simulink model "gm_dvfs_zed_simple_backup"  (R2025b)
settings: Solver=FixedStepDiscrete  StartTime=0.0  StopTime=10.0  FixedStep=0.1  RelTol=1e-3
libraries: simulink x6
settings Model: Creator=Vimal Rency  LastModifiedBy=Vimal Rency
settings OptimizationCC: BlockReduction=off  ConditionallyExecuteInputs=off
settings DebuggingCC: InheritedTsInSrcMsg=none

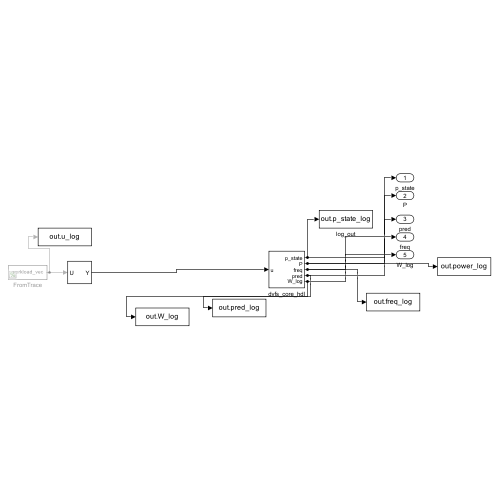
[thumbnail: Simulink's stored preview of the top-level diagram]
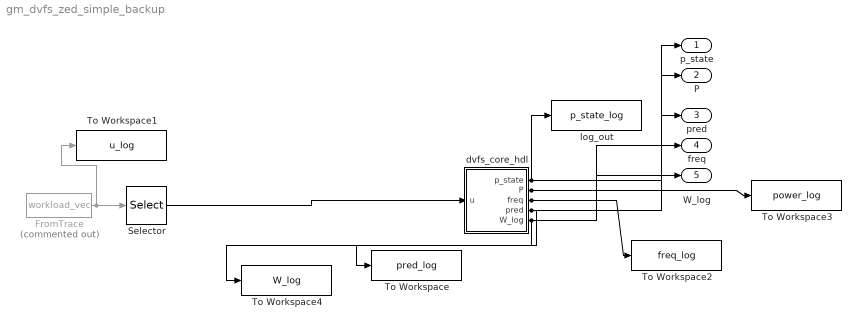
== system gm_dvfs_zed_simple_backup ==
  FromTrace : FromWorkspace  Commented=on  VariableName=workload_vec
  Selector : Selector  NumberOfDimensions=2  InputPortWidth=3  IndexOptions=Select all,Index vector (dialog)  Indices=[1 3],1  OutputSizes=1,1
  To Workspace : ToWorkspace  VariableName=pred_log  SampleTime=-1
  To Workspace1 : ToWorkspace  VariableName=u_log  SampleTime=-1
  To Workspace2 : ToWorkspace  VariableName=freq_log  SampleTime=-1
  To Workspace3 : ToWorkspace  VariableName=power_log  SampleTime=-1
  To Workspace4 : ToWorkspace  VariableName=W_log  SampleTime=-1
  dvfs_core_hdl : Subsystem
  log_out : ToWorkspace  VariableName=p_state_log  SampleTime=-1
  p_state : Outport
  P : Outport  Port=2
  pred : Outport  Port=3
  freq : Outport  Port=4
  W_log : Outport  Port=5
  wires:
  dvfs_core_hdl/5(W_log) -> To Workspace4/1, W_log/1
  dvfs_core_hdl/4(pred) -> To Workspace/1, pred/1
  dvfs_core_hdl/3(freq) -> To Workspace2/1, freq/1
  dvfs_core_hdl/2(P) -> To Workspace3/1, P/1
  dvfs_core_hdl/1(p_state) -> log_out/1, p_state/1
  Selector/1 -> dvfs_core_hdl/1(u)
  FromTrace/1 -> Selector/1, To Workspace1/1

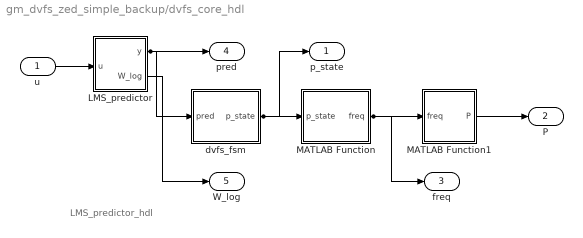
== system gm_dvfs_zed_simple_backup/dvfs_core_hdl ==
  note: LMS_predictor_hdl
  u : Inport  OutDataTypeStr=double  PortDimensions=1  SampleTime=0.1
  LMS_predictor : Subsystem
  MATLAB Function : Subsystem
  MATLAB Function1 : Subsystem
  dvfs_fsm : Subsystem
  p_state : Outport  SampleTime=0.1
  P : Outport  Port=2  SampleTime=0.1
  freq : Outport  Port=3  SampleTime=0.1
  pred : Outport  Port=4  SampleTime=0.1
  W_log : Outport  Port=5  SampleTime=0.1
  wires:
  u/1 -> LMS_predictor/1(u)
  dvfs_fsm/1(p_state) -> MATLAB Function/1(p_state), p_state/1
  LMS_predictor/1(y) -> dvfs_fsm/1(pred), pred/1
  LMS_predictor/2(W_log) -> W_log/1
  MATLAB Function/1(freq) -> MATLAB Function1/1(freq), freq/1
  MATLAB Function1/1(P) -> P/1

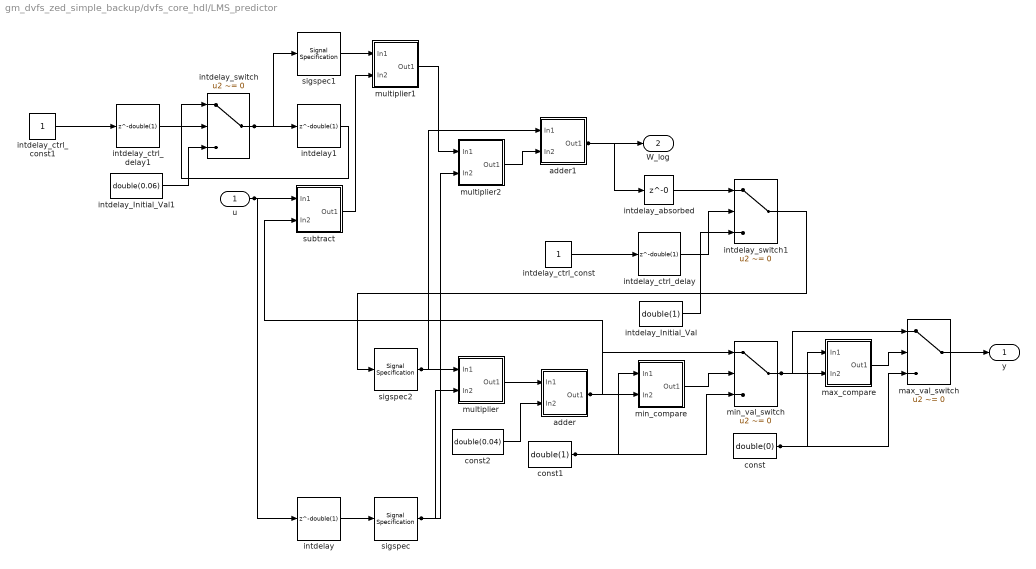
== system gm_dvfs_zed_simple_backup/dvfs_core_hdl/LMS_predictor ==
  u : Inport  OutDataTypeStr=double  PortDimensions=1  SampleTime=0.1
  adder : Subsystem
      mask Display: disp('NFP\nadd');
  adder1 : Subsystem
      mask Display: disp('NFP\nadd');
  const : Constant  Value=double(0)  VectorParams1D=off  OutDataTypeStr=double  SampleTime=0.1
  const1 : Constant  Value=double(1)  VectorParams1D=off  OutDataTypeStr=double  SampleTime=0.1
  const2 : Constant  Value=double(0.04)  VectorParams1D=off  OutDataTypeStr=double  SampleTime=0.1
  intdelay : Delay  DelayLength=double(1)  InitialCondition=0  SampleTime=0.1
  intdelay1 : Delay  DelayLength=double(1)  InitialCondition=0  SampleTime=0.1
  intdelay_Initial_Val : Constant  Value=double(1)  OutDataTypeStr=double  SampleTime=0.1
  intdelay_Initial_Val1 : Constant  Value=double(0.06)  OutDataTypeStr=double  SampleTime=0.1
  intdelay_absorbed : Delay  DelayLength=0
  intdelay_ctrl_const : Constant  OutDataTypeStr=boolean  SampleTime=0.1
  intdelay_ctrl_const1 : Constant  OutDataTypeStr=boolean  SampleTime=0.1
  intdelay_ctrl_delay : Delay  DelayLength=double(1)  InitialCondition=0  SampleTime=0.1
  intdelay_ctrl_delay1 : Delay  DelayLength=double(1)  InitialCondition=0  SampleTime=0.1
  intdelay_switch : Switch  Criteria=u2 ~= 0  Threshold=double(0)  OutDataTypeStr=double  SampleTime=0.1  SaturateOnIntegerOverflow=off  InputSameDT=off
  intdelay_switch1 : Switch  Criteria=u2 ~= 0  Threshold=double(0)  OutDataTypeStr=double  SampleTime=0.1  SaturateOnIntegerOverflow=off  InputSameDT=off
  max_compare : Subsystem
      mask Display: disp('NFP\nrelop');
  max_val_switch : Switch  Criteria=u2 ~= 0  Threshold=double(0)  OutDataTypeStr=double  SampleTime=0.1  SaturateOnIntegerOverflow=off  InputSameDT=off
  min_compare : Subsystem
      mask Display: disp('NFP\nrelop');
  min_val_switch : Switch  Criteria=u2 ~= 0  Threshold=double(0)  OutDataTypeStr=double  SampleTime=0.1  SaturateOnIntegerOverflow=off  InputSameDT=off
  multiplier : Subsystem
      mask Display: disp('NFP\nmul');
  multiplier1 : Subsystem
      mask Display: disp('NFP\nmul');
  multiplier2 : Subsystem
      mask Display: disp('NFP\nmul');
  sigspec : SignalSpecification  OutDataTypeStr=double  Dimensions=1
  sigspec1 : SignalSpecification  OutDataTypeStr=double  Dimensions=1
  sigspec2 : SignalSpecification  OutDataTypeStr=double  Dimensions=1
  subtract : Subsystem
      mask Display: disp('NFP\nadd');
  y : Outport  SampleTime=0.1
  W_log : Outport  Port=2  SampleTime=0.1
  wires:
  sigspec1/1 -> multiplier1/1(In1)
  u/1 -> intdelay/1, subtract/1(In1)
  multiplier1/1(Out1) -> multiplier2/1(In1)
  intdelay_ctrl_const1/1 -> intdelay_ctrl_delay1/1
  intdelay1/1 -> intdelay_switch/1
  sigspec2/1 -> adder1/1(In1), multiplier/1(In1)
  intdelay_ctrl_delay1/1 -> intdelay_switch/2
  intdelay_Initial_Val1/1 -> intdelay_switch/3
  intdelay_switch1/1 -> sigspec2/1
  intdelay_switch/1 -> sigspec1/1, intdelay1/1
  subtract/1(Out1) -> multiplier1/2(In2)
  intdelay/1 -> sigspec/1
  sigspec/1 -> multiplier/2(In2), multiplier2/2(In2)
  intdelay_ctrl_delay/1 -> intdelay_switch1/2
  multiplier2/1(Out1) -> adder1/2(In2)
  multiplier/1(Out1) -> adder/1(In1)
  const2/1 -> adder/2(In2)
  adder1/1(Out1) -> intdelay_absorbed/1, W_log/1
  intdelay_ctrl_const/1 -> intdelay_ctrl_delay/1
  adder/1(Out1) -> min_val_switch/1, min_compare/2(In2), subtract/2(In2)
  const1/1 -> min_val_switch/3, min_compare/1(In1)
  intdelay_absorbed/1 -> intdelay_switch1/1
  intdelay_Initial_Val/1 -> intdelay_switch1/3
  min_compare/1(Out1) -> min_val_switch/2
  min_val_switch/1 -> max_val_switch/1, max_compare/2(In2)
  const/1 -> max_val_switch/3, max_compare/1(In1)
  max_compare/1(Out1) -> max_val_switch/2
  max_val_switch/1 -> y/1

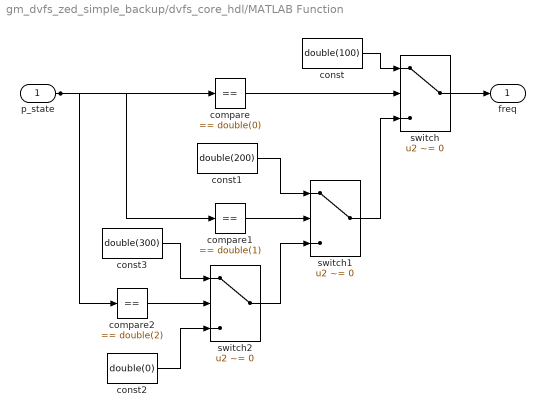
== system gm_dvfs_zed_simple_backup/dvfs_core_hdl/MATLAB Function ==
  p_state : Inport  OutDataTypeStr=uint8  PortDimensions=1  SampleTime=0.1
  compare : simulink/Logic and Bit Operations/Compare To Constant  relop===  const=double(0)  OutDataTypeStr=boolean
  compare1 : simulink/Logic and Bit Operations/Compare To Constant  relop===  const=double(1)  OutDataTypeStr=boolean
  compare2 : simulink/Logic and Bit Operations/Compare To Constant  relop===  const=double(2)  OutDataTypeStr=boolean
  const : Constant  Value=double(100)  VectorParams1D=off  OutDataTypeStr=double  SampleTime=0.1
  const1 : Constant  Value=double(200)  VectorParams1D=off  OutDataTypeStr=double  SampleTime=0.1
  const2 : Constant  Value=double(0)  VectorParams1D=off  OutDataTypeStr=double  SampleTime=0.1
  const3 : Constant  Value=double(300)  VectorParams1D=off  OutDataTypeStr=double  SampleTime=0.1
  switch : Switch  Criteria=u2 ~= 0  Threshold="fi(0,0,1,0,\"hex\",\"0\")"  OutDataTypeStr=double  SampleTime=0.1  SaturateOnIntegerOverflow=off  InputSameDT=off
  switch1 : Switch  Criteria=u2 ~= 0  Threshold="fi(0,0,1,0,\"hex\",\"0\")"  OutDataTypeStr=double  SampleTime=0.1  SaturateOnIntegerOverflow=off  InputSameDT=off
  switch2 : Switch  Criteria=u2 ~= 0  Threshold="fi(0,0,1,0,\"hex\",\"0\")"  OutDataTypeStr=double  SampleTime=0.1  SaturateOnIntegerOverflow=off  InputSameDT=off
  freq : Outport  SampleTime=0.1
  wires:
  const2/1 -> switch2/3
  p_state/1 -> compare1/1, compare/1, compare2/1
  const3/1 -> switch2/1
  switch2/1 -> switch1/3
  compare2/1 -> switch2/2
  compare/1 -> switch/2
  const1/1 -> switch1/1
  compare1/1 -> switch1/2
  const/1 -> switch/1
  switch1/1 -> switch/3
  switch/1 -> freq/1

== system gm_dvfs_zed_simple_backup/dvfs_core_hdl/MATLAB Function1 ==
  freq : Inport  OutDataTypeStr=double  PortDimensions=1  SampleTime=0.1
  gain : Subsystem
      mask Display: disp('NFP\nmul');
  gain_const : Constant  Value=double(0.01)  OutDataTypeStr=double  SampleTime=0.1
  P : Outport  SampleTime=0.1
  wires:
  gain/1(Out1) -> P/1
  gain_const/1 -> gain/1(In1)
  freq/1 -> gain/2(In2)

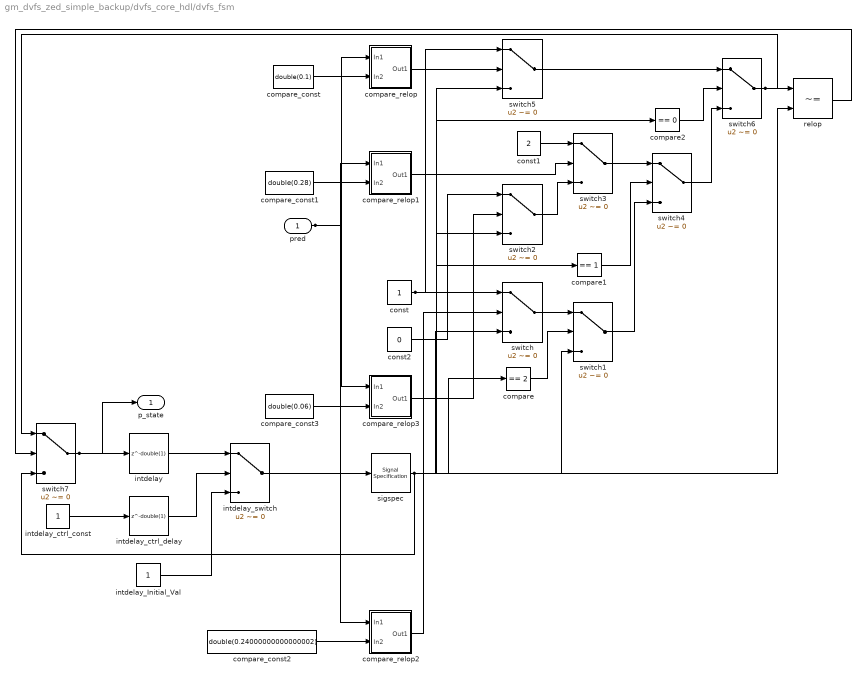
== system gm_dvfs_zed_simple_backup/dvfs_core_hdl/dvfs_fsm ==
  pred : Inport  OutDataTypeStr=double  PortDimensions=1  SampleTime=0.1
  compare : simulink/Logic and Bit Operations/Compare To Constant  relop===  const=2  OutDataTypeStr=boolean
  compare1 : simulink/Logic and Bit Operations/Compare To Constant  relop===  const=1  OutDataTypeStr=boolean
  compare2 : simulink/Logic and Bit Operations/Compare To Constant  relop===  const=0  OutDataTypeStr=boolean
  compare_const : Constant  Value=double(0.1)  OutDataTypeStr=double  SampleTime=0.1
  compare_const1 : Constant  Value=double(0.28)  OutDataTypeStr=double  SampleTime=0.1
  compare_const2 : Constant  Value=double(0.24000000000000002)  OutDataTypeStr=double  SampleTime=0.1
  compare_const3 : Constant  Value=double(0.06)  OutDataTypeStr=double  SampleTime=0.1
  compare_relop : Subsystem
      mask Display: disp('NFP\nrelop');
  compare_relop1 : Subsystem
      mask Display: disp('NFP\nrelop');
  compare_relop2 : Subsystem
      mask Display: disp('NFP\nrelop');
  compare_relop3 : Subsystem
      mask Display: disp('NFP\nrelop');
  const : Constant  VectorParams1D=off  OutDataTypeStr=uint8  SampleTime=0.1
  const1 : Constant  Value=2  VectorParams1D=off  OutDataTypeStr=uint8  SampleTime=0.1
  const2 : Constant  Value=0  VectorParams1D=off  OutDataTypeStr=uint8  SampleTime=0.1
  intdelay : Delay  DelayLength=double(1)  InitialCondition=0  SampleTime=0.1
  intdelay_Initial_Val : Constant  OutDataTypeStr=uint8  SampleTime=0.1
  intdelay_ctrl_const : Constant  OutDataTypeStr=boolean  SampleTime=0.1
  intdelay_ctrl_delay : Delay  DelayLength=double(1)  InitialCondition=0  SampleTime=0.1
  intdelay_switch : Switch  Criteria=u2 ~= 0  Threshold=double(0)  OutDataTypeStr=uint8  SampleTime=0.1  SaturateOnIntegerOverflow=off  InputSameDT=off
  relop : RelationalOperator  Operator=~=  OutDataTypeStr=boolean  SampleTime=0.1  InputSameDT=off
  sigspec : SignalSpecification  OutDataTypeStr=uint8  Dimensions=1
  switch{,1..7} (8 alike) : Switch  Criteria=u2 ~= 0  Threshold="fi(0,0,1,0,\"hex\",\"0\")"  OutDataTypeStr=uint8  SampleTime=0.1  SaturateOnIntegerOverflow=off  InputSameDT=off
  p_state : Outport  SampleTime=0.1
  wires:
  switch7/1 -> p_state/1, intdelay/1
  intdelay_Initial_Val/1 -> intdelay_switch/3
  intdelay_ctrl_const/1 -> intdelay_ctrl_delay/1
  sigspec/1 -> switch7/3, switch1/3, compare2/1, relop/2, compare1/1, switch2/3, switch/3, compare/1, switch5/3
  compare_const/1 -> compare_relop/2(In2)
  intdelay/1 -> intdelay_switch/1
  compare_const1/1 -> compare_relop1/2(In2)
  intdelay_ctrl_delay/1 -> intdelay_switch/2
  pred/1 -> compare_relop1/1(In1), compare_relop/1(In1), compare_relop2/1(In1), compare_relop3/1(In1)
  compare_relop2/1(Out1) -> switch/2
  compare_const3/1 -> compare_relop3/2(In2)
  intdelay_switch/1 -> sigspec/1
  switch1/1 -> switch4/3
  compare_const2/1 -> compare_relop2/2(In2)
  const1/1 -> switch3/1
  compare_relop/1(Out1) -> switch5/2
  compare_relop1/1(Out1) -> switch3/2
  const/1 -> switch5/1, switch/1
  const2/1 -> switch2/1
  compare_relop3/1(Out1) -> switch2/2
  switch5/1 -> switch6/1
  switch2/1 -> switch3/3
  switch/1 -> switch1/1
  compare/1 -> switch1/2
  switch3/1 -> switch4/1
  compare1/1 -> switch4/2
  compare2/1 -> switch6/2
  switch4/1 -> switch6/3
  switch6/1 -> switch7/1, relop/1
  relop/1 -> switch7/2

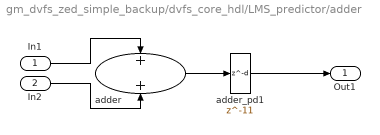
== system gm_dvfs_zed_simple_backup/dvfs_core_hdl/LMS_predictor/adder ==
  In1 : Inport
  In2 : Inport  Port=2
  adder : Sum  OutDataTypeStr=double  SampleTime=0.1
  adder_pd1 : Delay  DelayLength=11
  Out1 : Outport
  wires:
  In1/1 -> adder/1
  In2/1 -> adder/2
  adder/1 -> adder_pd1/1
  adder_pd1/1 -> Out1/1

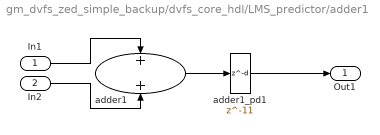
== system gm_dvfs_zed_simple_backup/dvfs_core_hdl/LMS_predictor/adder1 ==
  In1 : Inport
  In2 : Inport  Port=2
  adder1 : Sum  OutDataTypeStr=double  SampleTime=0.1
  adder1_pd1 : Delay  DelayLength=11
  Out1 : Outport
  wires:
  In1/1 -> adder1/1
  In2/1 -> adder1/2
  adder1/1 -> adder1_pd1/1
  adder1_pd1/1 -> Out1/1

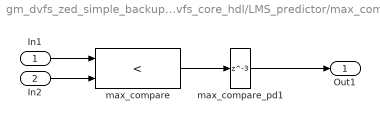
== system gm_dvfs_zed_simple_backup/dvfs_core_hdl/LMS_predictor/max_compare ==
  In1 : Inport
  In2 : Inport  Port=2
  max_compare : RelationalOperator  Operator=<  OutDataTypeStr=boolean  SampleTime=0.1
  max_compare_pd1 : Delay  DelayLength=3
  Out1 : Outport
  wires:
  In1/1 -> max_compare/1
  In2/1 -> max_compare/2
  max_compare/1 -> max_compare_pd1/1
  max_compare_pd1/1 -> Out1/1

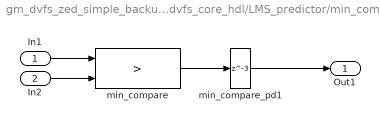
== system gm_dvfs_zed_simple_backup/dvfs_core_hdl/LMS_predictor/min_compare ==
  In1 : Inport
  In2 : Inport  Port=2
  min_compare : RelationalOperator  Operator=>  OutDataTypeStr=boolean  SampleTime=0.1
  min_compare_pd1 : Delay  DelayLength=3
  Out1 : Outport
  wires:
  In1/1 -> min_compare/1
  In2/1 -> min_compare/2
  min_compare/1 -> min_compare_pd1/1
  min_compare_pd1/1 -> Out1/1

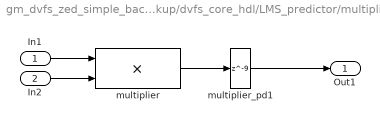
== system gm_dvfs_zed_simple_backup/dvfs_core_hdl/LMS_predictor/multiplier ==
  In1 : Inport
  In2 : Inport  Port=2
  multiplier : Product  Inputs=**  OutDataTypeStr=double  SampleTime=0.1
  multiplier_pd1 : Delay  DelayLength=9
  Out1 : Outport
  wires:
  In1/1 -> multiplier/1
  In2/1 -> multiplier/2
  multiplier/1 -> multiplier_pd1/1
  multiplier_pd1/1 -> Out1/1

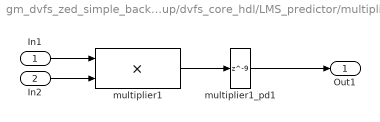
== system gm_dvfs_zed_simple_backup/dvfs_core_hdl/LMS_predictor/multiplier1 ==
  In1 : Inport
  In2 : Inport  Port=2
  multiplier1 : Product  Inputs=**  OutDataTypeStr=double  SampleTime=0.1
  multiplier1_pd1 : Delay  DelayLength=9
  Out1 : Outport
  wires:
  In1/1 -> multiplier1/1
  In2/1 -> multiplier1/2
  multiplier1/1 -> multiplier1_pd1/1
  multiplier1_pd1/1 -> Out1/1

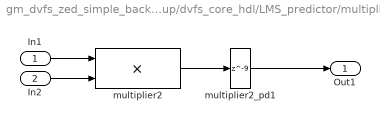
== system gm_dvfs_zed_simple_backup/dvfs_core_hdl/LMS_predictor/multiplier2 ==
  In1 : Inport
  In2 : Inport  Port=2
  multiplier2 : Product  Inputs=**  OutDataTypeStr=double  SampleTime=0.1
  multiplier2_pd1 : Delay  DelayLength=9
  Out1 : Outport
  wires:
  In1/1 -> multiplier2/1
  In2/1 -> multiplier2/2
  multiplier2/1 -> multiplier2_pd1/1
  multiplier2_pd1/1 -> Out1/1

== system gm_dvfs_zed_simple_backup/dvfs_core_hdl/LMS_predictor/subtract ==
  In1 : Inport
  In2 : Inport  Port=2
  subtract : Sum  Inputs=+-  OutDataTypeStr=double  SampleTime=0.1
  subtract_pd1 : Delay  DelayLength=11
  Out1 : Outport
  wires:
  In1/1 -> subtract/1
  In2/1 -> subtract/2
  subtract/1 -> subtract_pd1/1
  subtract_pd1/1 -> Out1/1

== system gm_dvfs_zed_simple_backup/dvfs_core_hdl/MATLAB Function1/gain ==
  In1 : Inport
  In2 : Inport  Port=2
  gain : Product  Inputs=**  OutDataTypeStr=double  SampleTime=0.1
  gain_pd1 : Delay  DelayLength=9
  Out1 : Outport
  wires:
  In1/1 -> gain/1
  In2/1 -> gain/2
  gain/1 -> gain_pd1/1
  gain_pd1/1 -> Out1/1

== system gm_dvfs_zed_simple_backup/dvfs_core_hdl/dvfs_fsm/compare_relop ==
  In1 : Inport
  In2 : Inport  Port=2
  compare_relop : RelationalOperator  OutDataTypeStr=boolean  SampleTime=0.1
  compare_relop_pd1 : Delay  DelayLength=3
  Out1 : Outport
  wires:
  In1/1 -> compare_relop/1
  In2/1 -> compare_relop/2
  compare_relop/1 -> compare_relop_pd1/1
  compare_relop_pd1/1 -> Out1/1

== system gm_dvfs_zed_simple_backup/dvfs_core_hdl/dvfs_fsm/compare_relop1 ==
  In1 : Inport
  In2 : Inport  Port=2
  compare_relop1 : RelationalOperator  OutDataTypeStr=boolean  SampleTime=0.1
  compare_relop1_pd1 : Delay  DelayLength=3
  Out1 : Outport
  wires:
  In1/1 -> compare_relop1/1
  In2/1 -> compare_relop1/2
  compare_relop1/1 -> compare_relop1_pd1/1
  compare_relop1_pd1/1 -> Out1/1

== system gm_dvfs_zed_simple_backup/dvfs_core_hdl/dvfs_fsm/compare_relop2 ==
  In1 : Inport
  In2 : Inport  Port=2
  compare_relop2 : RelationalOperator  Operator=<  OutDataTypeStr=boolean  SampleTime=0.1
  compare_relop2_pd1 : Delay  DelayLength=3
  Out1 : Outport
  wires:
  In1/1 -> compare_relop2/1
  In2/1 -> compare_relop2/2
  compare_relop2/1 -> compare_relop2_pd1/1
  compare_relop2_pd1/1 -> Out1/1

== system gm_dvfs_zed_simple_backup/dvfs_core_hdl/dvfs_fsm/compare_relop3 ==
  In1 : Inport
  In2 : Inport  Port=2
  compare_relop3 : RelationalOperator  Operator=<  OutDataTypeStr=boolean  SampleTime=0.1
  compare_relop3_pd1 : Delay  DelayLength=3
  Out1 : Outport
  wires:
  In1/1 -> compare_relop3/1
  In2/1 -> compare_relop3/2
  compare_relop3/1 -> compare_relop3_pd1/1
  compare_relop3_pd1/1 -> Out1/1
